simulink model "verificaModelloLTI"  (R2021a)
settings: Solver=FixedStepAuto  StartTime=0.0  StopTime=25  FixedStep=Tc  RelTol=1e-3
values from neighbouring files (symbols this model uses):
  Tc = 0.01    [esercizio2.m]
settings Model: Creator=Giorgio  LastModifiedBy=Giorgio

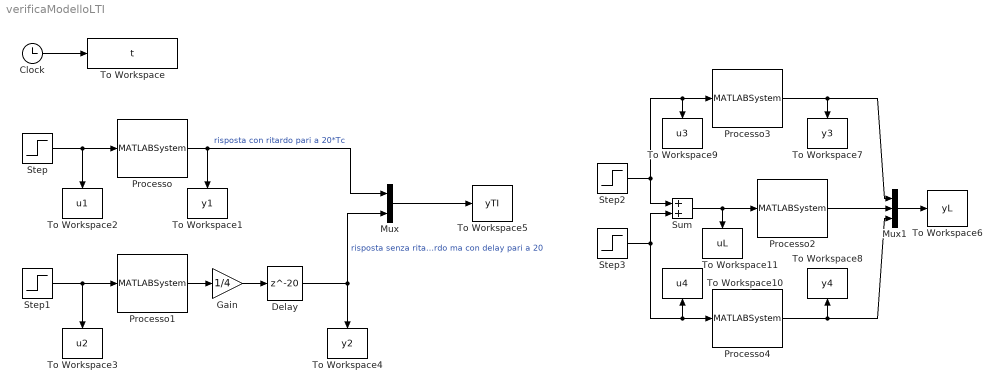
== system verificaModelloLTI ==
  Clock : Clock
  Delay : Delay  DelayLength=20
  Gain : Gain  Gain=1/4
  Mux : Mux  Inputs=2
  Mux1 : Mux  Inputs=3
  Processo{,1..4} (5 alike) : MATLABSystem  System=linSysObj  SimulateUsing=Interpreted execution
      mask Type: linSysObj
      mask Display:
      | disp('Black box');
      | port_label('input',1,'u');
      | port_label('output',1,'y');
  Step : Step  Time=20*Tc  SampleTime=0
  Step1 : Step  Time=0  After=4  SampleTime=0
  Step2 : Step  Time=0  SampleTime=0
  Step3 : Step  Time=0  After=2  SampleTime=0
  Sum : Sum
  To Workspace : ToWorkspace  VariableName=t  SampleTime=-1
      settings: Save2DSignal=2-D array (concatenate along first dimension)
  To Workspace1 : ToWorkspace  VariableName=y1  SampleTime=-1
      settings: Save2DSignal=2-D array (concatenate along first dimension)
  To Workspace10 : ToWorkspace  VariableName=u4  SampleTime=-1
      settings: Save2DSignal=2-D array (concatenate along first dimension)
  To Workspace11 : ToWorkspace  VariableName=uL  SampleTime=-1
      settings: Save2DSignal=2-D array (concatenate along first dimension)
  To Workspace2 : ToWorkspace  VariableName=u1  SampleTime=-1
      settings: Save2DSignal=2-D array (concatenate along first dimension)
  To Workspace3 : ToWorkspace  VariableName=u2  SampleTime=-1
      settings: Save2DSignal=2-D array (concatenate along first dimension)
  To Workspace4 : ToWorkspace  VariableName=y2  SampleTime=-1
      settings: Save2DSignal=2-D array (concatenate along first dimension)
  To Workspace5 : ToWorkspace  VariableName=yTI  SampleTime=-1
      settings: Save2DSignal=2-D array (concatenate along first dimension)
  To Workspace6 : ToWorkspace  VariableName=yL  SampleTime=-1
      settings: Save2DSignal=2-D array (concatenate along first dimension)
  To Workspace7 : ToWorkspace  VariableName=y3  SampleTime=-1
      settings: Save2DSignal=2-D array (concatenate along first dimension)
  To Workspace8 : ToWorkspace  VariableName=y4  SampleTime=-1
      settings: Save2DSignal=2-D array (concatenate along first dimension)
  To Workspace9 : ToWorkspace  VariableName=u3  SampleTime=-1
      settings: Save2DSignal=2-D array (concatenate along first dimension)
  wires:
  Clock/1 -> To Workspace/1
  Step/1 -> Processo/1, To Workspace2/1
  Step1/1 -> Processo1/1, To Workspace3/1
  Processo1/1 -> Gain/1
  Processo/1 -> Mux/1, To Workspace1/1  "risposta con ritardo pari a 20*Tc"
  Gain/1 -> Delay/1
  Delay/1 -> Mux/2, To Workspace4/1  "risposta senza ritardo ma con delay pari a 20"
  Mux/1 -> To Workspace5/1
  Step2/1 -> To Workspace9/1, Processo3/1, Sum/1
  Step3/1 -> Sum/2, Processo4/1, To Workspace10/1
  Sum/1 -> To Workspace11/1, Processo2/1
  Processo2/1 -> Mux1/2
  Processo3/1 -> Mux1/1, To Workspace7/1
  Processo4/1 -> To Workspace8/1, Mux1/3
  Mux1/1 -> To Workspace6/1
